simulink model "TrailerSoftware"  (R2019b)
settings: Solver=FixedStepDiscrete  StartTime=0.0  StopTime=inf  FixedStep=update  RelTol=1e-3  EnableMultiTasking=on
values from neighbouring files (symbols this model uses):
  countmax1 = 2500    [ProductionMfile.m]
  countmax2 = 2500    [ProductionMfile.m]
  HeaterIntGain = .0008    (= 0.0008)    [ProductionMfile.m]
  HeatGain = 10    [ProductionMfile.m]
  Intll = 0    [ProductionMfile.m]
  MaxCondPressure = 350    [ProductionMfile.m]
  MinSP = 1    [ProductionMfile.m]
  PostGain100 = 0.0002    [ProductionMfile.m]
  PostGain150 = 0.0005    [ProductionMfile.m]
  PostGain200 = 0.0004    [ProductionMfile.m]
  PostGain300 = 0.0008    [ProductionMfile.m]
  PostInit150 = 12    [ProductionMfile.m]
  PostIntulC = 65    [ProductionMfile.m]
  PostPGain = 0    [ProductionMfile.m]
  PreGain100 = 0.0005    [ProductionMfile.m]
  PreGain150 = 0.0005    [ProductionMfile.m]
  PreGain200 = 0.0003    [ProductionMfile.m]
  PreGain300 = 0.0008    [ProductionMfile.m]
  PreInit150 = 30    [ProductionMfile.m]
  PreIntulC = 65    [ProductionMfile.m]
  PreIntulDH = 65    [ProductionMfile.m]
  PrePGain = 0    [ProductionMfile.m]
  SatPress = [10 20 30 40 50 60 70 80 90 100 110 120 130 140 150 160 170      180 190 200 210 220 230 240 250 260 270 280 290 300 310 320 330      340 350 360 370 380 390 400 410 420 430 440 450 460 470 480 490      500]    [ProductionMfile.m]
  SatTemp = [-29.497 -2.4046 15.401 29.047 40.267 49.88 58.338 65.922 72.819      79.159 85.037 90.526 95.68 100.55 105.16 109.54 113.73 117.73 121.57      125.26 128.82 132.25 135.56 138.77 141.88 144.89 147.82 150.67 153.44      156.15 158.78 161.35 163.85 166.3 168.7 171.04 173.33 175.58 177.77      179.93 182.04 184.11 186.14 188.14 190.09 192.01 193.9 195.75 197.58      199.37]    [ProductionMfile.m]
  SHGain = 2    [ProductionMfile.m]
  SizeCANMatrix = 80    [ProductionMfile.m]
  SizeCOBIDVector = 10    [ProductionMfile.m]
  update = 0.002    [ProductionMfile.m]
undefined symbols (not defined in the file or in its folder): DiscIntNeverNeededParam, PostDGain, PreDGain, Ratio100, Ratio150, Ratio200, Ratio300
libraries: simulink x60, c2837xDlib x35, xpcutilitieslib x24, c2802xlib x8, c280xlib x7, etargetslib x4, svdutilitieslib x2, c2000lib x1
(part 1 of 8)
settings Model: SimulationMode=external  ExtModeTrigDuration=8  Creator=steve  LastModifiedBy=steve
settings SolverCC: AutoInsertRateTranBlk=on
settings DataIOCC: SaveOutput=off  SignalLogging=off  DSMLogging=off  SaveTime=off  ReturnWorkspaceOutputs=off
settings OptimizationCC: DefaultUnderspecifiedDataType=single  EnhancedBackFolding=on  PassReuseOutputArgsAs=Individual arguments  MaxStackSize=1024  OptimizeBlockOrder=speed  DifferentSizesBufferReuse=on  OptimizationCustomize=off  EfficientTunableParamExpr=on
settings DebuggingCC: ParameterTunabilityLossMsg=error
settings HardwareCC: ProdBitPerChar=16  ProdBitPerInt=16  ProdBitPerPointer=32  ProdBitPerSizeT=32  ProdBitPerPtrDiffT=32  ProdLargestAtomicInteger=Integer  ProdLargestAtomicFloat=None  ProdWordSize=16  ProdLongLongMode=on  ProdHWDeviceType=Texas Instruments->C2000
settings SFSimCC: SimCustomSourceCode=src/DisplayFunction.c  SimCustomHeaderCode="#include \"DisplayFunction.h\""  SimUserIncludeDirs=include  MATLABDynamicMemAlloc=off  DefaultCustomCodeFunctionArrayLayout=Row-major  CustomCodeUndefinedFunction=UseInterfaceOnly
settings RTWCC: SystemTargetFile=ert.tlc  HardwareBoard=TI Delfino F28379D LaunchPad  TLCOptions=-aInlineSetEventsForThisBaseRateFcn=TLC_FALSE -aSuppressMultiTaskScheduler=TLC_FALSE -aRateBasedStepFcn=1  TemplateMakefile=ert_default_tmf  Toolchain=Texas Instruments Code Composer Studio (C2000)  IncludeHyperlinkInReport=on
settings CodeAppCC: ForceParamTrailComments=on  IgnoreCustomStorageClasses=off  OperatorAnnotations=on  SimulinkDataObjDesc=on  SFDataObjDesc=on  InsertBlockDesc=on
settings ERTTargetCC: CodeReplacementLibrary=TI C28x  ExtMode=on  ExtModeTransport=3  ExtModeStaticAllocSize=10000  ExtModeMexArgs='127.0.0.1' 0 17725

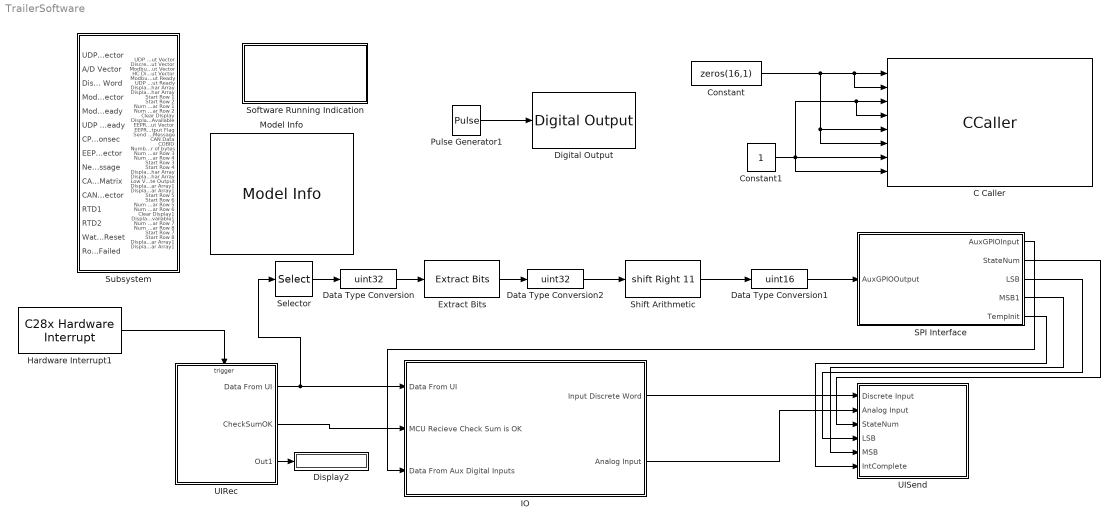
== system TrailerSoftware ==
  C Caller : CCaller  FunctionName=DisplayFunction  PortSpecificationStruct="%)30     .    > X   8    (     @         %    \"     @    !     0         %  0 \"0    $    _    07)G3F%M90  4&]R=$YA;64 4V-O<&4     26YD97@     5'EP90      4VEZ90      27-';&]B86P   X   !     !@    @    $          4    (     0    L    !         !     +    1&ES<&QA>5)O=S$       X   !     !@    @    $          4    (     0    L    !         !     +    1&ES<&QA>5)O=S$       X    X    !@    @    $     ...(+4615 chars)"
  Constant : Constant  Value=zeros(16,1)  OutDataTypeStr=uint8
  Constant1 : Constant  OutDataTypeStr=uint8
  Data Type Conversion : DataTypeConversion  OutDataTypeStr=uint32
  Data Type Conversion1 : DataTypeConversion  OutDataTypeStr=uint16
  Data Type Conversion2 : DataTypeConversion  OutDataTypeStr=uint32
  Digital Output : c2837xDlib/Digital Output  GPIO_Number=GPIO56~GPIO63  GPIO_Bit0=off  GPIO_BIT0_Toggle=off  GPIO_Bit1=off  GPIO_BIT1_Toggle=off  GPIO_Bit2=off  GPIO_BIT2_Toggle=off  GPIO_Bit3=off  GPIO_BIT3_Toggle=off  GPIO_Bit4=off  GPIO_BIT4_Toggle=off  GPIO_Bit5=off  GPIO_BIT5_Toggle=off  GPIO_Bit6=off  GPIO_BIT6_Toggle=off  GPIO_Bit7=on  GPIO_BIT7_Toggle=off
      settings: SourceProductName=Embedded Coder Support Package for Texas Instruments C2000 Processors  SourceProductBaseCode=TIC2000
  Display2 : Display
  Extract Bits : simulink/Logic and Bit Operations/Extract Bits  bitsToExtract=Range of bits  numBits=8  bitIdxRange=[11 18]  outScalingMode=Preserve fixed-point scaling
      settings: SourceProductName=Simulink
  Hardware Interrupt1 : c2000lib/Scheduling/C28x Hardware Interrupt  irqnumbers=[9]  pienumbers=[3]  irqpriorities=[30]  irqpreempts=[1]  showinput=off  dspchiptype=C280X
      settings: SourceProductName=Embedded Coder Support Package for Texas Instruments C2000 Processors  SourceProductBaseCode=TIC2000
  IO : Subsystem
  Model Info : simulink/Model-Wide Utilities/Model Info  Frame=on  DisplayStringWithTags=|  HorizontalTextAlignment=Center  LeftAlignmentValue=0.5
      | Model Info
      | %<Creator>
      | %<ModifiedBy>
      | %<ModelVersion>
      | %<Description>
      | %<LastModifiedBy>
      | %<LastModificationDate>
  Pulse Generator1 : DiscretePulseGenerator  SampleTime=update  VectorParams1D=off
  SPI Interface : Subsystem
  Selector : Selector  InputPortWidth=4  IndexOptions=Index vector (dialog)  Indices=[1]  OutputSizes=1
  Shift Arithmetic : ArithShift  BitShiftNumber=11  BitShiftDirection=Right
  Software Running Indication : Subsystem
  Subsystem : Subsystem
  UIRec : Subsystem
  UISend : Subsystem  TreatAsAtomicUnit=on  SystemSampleTime=.01
  wires:
  IO/1(Input Discrete Word) -> UISend/1(" Discrete Input")
  UIRec/2(CheckSumOK) -> IO/2(MCU Recieve Check Sum is OK)
  UIRec/1(Data From UI) -> Selector/1, IO/1(Data From UI)
  Pulse Generator1/1 -> Digital Output/1
  SPI Interface/1(AuxGPIOInput) -> IO/3(Data From Aux Digital Inputs)
  IO/2(Analog Input) -> UISend/2(Analog Input)
  UIRec/3(Out1) -> Display2/1
  Selector/1 -> Data Type Conversion/1
  Data Type Conversion/1 -> Extract Bits/1
  Extract Bits/1 -> Data Type Conversion2/1
  Shift Arithmetic/1 -> Data Type Conversion1/1
  Data Type Conversion1/1 -> SPI Interface/1(AuxGPIOOutput)
  Data Type Conversion2/1 -> Shift Arithmetic/1
  Hardware Interrupt1/1 -> UIRec/Trigger
  SPI Interface/2(StateNum) -> UISend/3(StateNum)
  SPI Interface/3(LSB) -> UISend/4(LSB)
  SPI Interface/4(MSB1) -> UISend/5(MSB)
  SPI Interface/5(TempInit) -> UISend/6(IntComplete)
  Constant/1 -> C Caller/6, C Caller/5, C Caller/2, C Caller/1
  Constant1/1 -> C Caller/4, C Caller/3, C Caller/8, C Caller/7

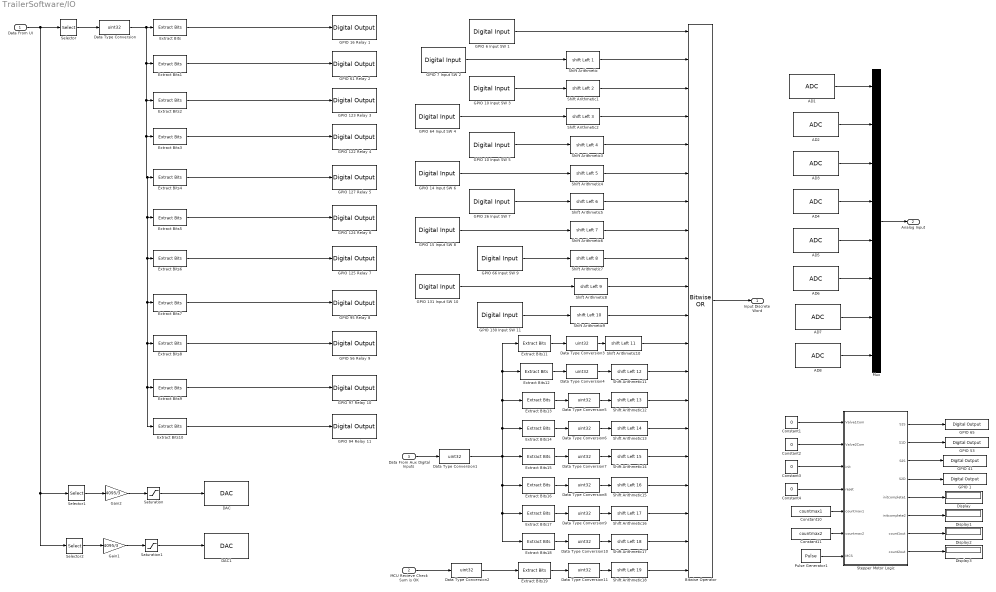
== system TrailerSoftware/IO ==
  Data From UI : Inport
  MCU Recieve Check Sum is OK : Inport  Port=2
  Data From Aux Digital Inputs : Inport  Port=3  OutDataTypeStr=uint16
  AD1 : c2802xlib/ADC  blkParamProc=C2000_Type4  ADCModule=C  samplingMode=Single sample mode  ADCResolution=12-bit (Single-ended input)  useSOC1=SOC0  useSOC2=SOC0_SOC1  SOCAcquisitionWindow=15  SOCTriggerSource=Software  SOCInterruptTrigger=No ADCINT  Ts=update  dType=uint16  postInterrupt=off  interruptSel=ADCINT1  ADCINTContinuous=on  endma=off  chdma=1  conv1=ADCINA0  conv2=ADCINA0 and ADCINB0  conv1_Type4=ADCIN3  conv2_Type4=ADCIN0 and ADCIN1
      settings: SourceProductName=Embedded Coder Support Package for Texas Instruments C2000 Processors
  AD2 : c2802xlib/ADC  blkParamProc=C2000_Type4  ADCModule=B  samplingMode=Single sample mode  ADCResolution=12-bit (Single-ended input)  useSOC1=SOC1  useSOC2=SOC0_SOC1  SOCAcquisitionWindow=15  SOCTriggerSource=Software  SOCInterruptTrigger=No ADCINT  Ts=update  dType=uint16  postInterrupt=off  interruptSel=ADCINT1  ADCINTContinuous=on  endma=off  chdma=1  conv1=ADCINA0  conv2=ADCINA0 and ADCINB0  conv1_Type4=ADCIN3  conv2_Type4=ADCIN0 and ADCIN1
      settings: SourceProductName=Embedded Coder Support Package for Texas Instruments C2000 Processors
  AD3 : c2802xlib/ADC  blkParamProc=C2000_Type4  ADCModule=A  samplingMode=Single sample mode  ADCResolution=12-bit (Single-ended input)  useSOC1=SOC2  useSOC2=SOC0_SOC1  SOCAcquisitionWindow=15  SOCTriggerSource=Software  SOCInterruptTrigger=No ADCINT  Ts=update  dType=uint16  postInterrupt=off  interruptSel=ADCINT1  ADCINTContinuous=on  endma=off  chdma=1  conv1=ADCINA0  conv2=ADCINA0 and ADCINB0  conv1_Type4=ADCIN3  conv2_Type4=ADCIN0 and ADCIN1
      settings: SourceProductName=Embedded Coder Support Package for Texas Instruments C2000 Processors
  AD4 : c2802xlib/ADC  blkParamProc=C2000_Type4  ADCModule=C  samplingMode=Single sample mode  ADCResolution=12-bit (Single-ended input)  useSOC1=SOC3  useSOC2=SOC0_SOC1  SOCAcquisitionWindow=15  SOCTriggerSource=Software  SOCInterruptTrigger=No ADCINT  Ts=update  dType=uint16  postInterrupt=off  interruptSel=ADCINT1  ADCINTContinuous=on  endma=off  chdma=1  conv1=ADCINA0  conv2=ADCINA0 and ADCINB0  conv1_Type4=ADCIN2  conv2_Type4=ADCIN0 and ADCIN1
      settings: SourceProductName=Embedded Coder Support Package for Texas Instruments C2000 Processors
  AD5 : c2802xlib/ADC  blkParamProc=C2000_Type4  ADCModule=B  samplingMode=Single sample mode  ADCResolution=12-bit (Single-ended input)  useSOC1=SOC5  useSOC2=SOC0_SOC1  SOCAcquisitionWindow=15  SOCTriggerSource=Software  SOCInterruptTrigger=No ADCINT  Ts=update  dType=uint16  postInterrupt=off  interruptSel=ADCINT1  ADCINTContinuous=on  endma=off  chdma=1  conv1=ADCINA0  conv2=ADCINA0 and ADCINB0  conv1_Type4=ADCIN2  conv2_Type4=ADCIN0 and ADCIN1
      settings: SourceProductName=Embedded Coder Support Package for Texas Instruments C2000 Processors
  AD6 : c2802xlib/ADC  blkParamProc=C2000_Type4  ADCModule=A  samplingMode=Single sample mode  ADCResolution=12-bit (Single-ended input)  useSOC1=SOC5  useSOC2=SOC0_SOC1  SOCAcquisitionWindow=15  SOCTriggerSource=Software  SOCInterruptTrigger=No ADCINT  Ts=update  dType=uint16  postInterrupt=off  interruptSel=ADCINT1  ADCINTContinuous=on  endma=off  chdma=1  conv1=ADCINA0  conv2=ADCINA0 and ADCINB0  conv1_Type4=ADCIN2  conv2_Type4=ADCIN0 and ADCIN1
      settings: SourceProductName=Embedded Coder Support Package for Texas Instruments C2000 Processors
  AD7 : c2802xlib/ADC  blkParamProc=C2000_Type4  ADCModule=B  samplingMode=Single sample mode  ADCResolution=12-bit (Single-ended input)  useSOC1=SOC6  useSOC2=SOC0_SOC1  SOCAcquisitionWindow=15  SOCTriggerSource=Software  SOCInterruptTrigger=No ADCINT  Ts=update  dType=uint16  postInterrupt=off  interruptSel=ADCINT1  ADCINTContinuous=on  endma=off  chdma=1  conv1=ADCINA0  conv2=ADCINA0 and ADCINB0  conv1_Type4=ADCIN4  conv2_Type4=ADCIN0 and ADCIN1
      settings: SourceProductName=Embedded Coder Support Package for Texas Instruments C2000 Processors
  AD8 : c2802xlib/ADC  blkParamProc=C2000_Type4  ADCModule=C  samplingMode=Single sample mode  ADCResolution=12-bit (Single-ended input)  useSOC1=SOC7  useSOC2=SOC0_SOC1  SOCAcquisitionWindow=15  SOCTriggerSource=Software  SOCInterruptTrigger=No ADCINT  Ts=update  dType=uint16  postInterrupt=off  interruptSel=ADCINT1  ADCINTContinuous=on  endma=off  chdma=1  conv1=ADCINA0  conv2=ADCINA0 and ADCINB0  conv1_Type4=ADCIN5  conv2_Type4=ADCIN0 and ADCIN1
      settings: SourceProductName=Embedded Coder Support Package for Texas Instruments C2000 Processors
  Bitwise Operator : simulink/Logic and Bit Operations/Bitwise Operator  logicop=OR  UseBitMask=off  NumInputPorts=20  BitMask=bin2dec('000000000000')  BitMaskRealWorld=Stored Integer
  Constant{1..4} (4 alike) : Constant  Value=0
  Constant10 : Constant  Value=countmax1
  Constant11 : Constant  Value=countmax2
  DAC : c2837xDlib/DAC  channel=A  saturate=on
      settings: SourceProductName=Embedded Coder Support Package for Texas Instruments C2000 Processors  SourceProductBaseCode=TIC2000
  DAC1 : c2837xDlib/DAC  channel=B  saturate=on
      settings: SourceProductName=Embedded Coder Support Package for Texas Instruments C2000 Processors  SourceProductBaseCode=TIC2000
  Data Type Conversion{,1..11} (12 alike) : DataTypeConversion  OutDataTypeStr=uint32
  Display{,1..3} (4 alike) : Display
  Extract Bits : simulink/Logic and Bit Operations/Extract Bits  bitsToExtract=Range of bits  numBits=8  bitIdxRange=[0]  outScalingMode=Treat bit field as an integer
      settings: SourceProductName=Simulink
  Extract Bits1 : simulink/Logic and Bit Operations/Extract Bits  bitsToExtract=Range of bits  numBits=8  bitIdxRange=[1]  outScalingMode=Treat bit field as an integer
      settings: SourceProductName=Simulink
  Extract Bits10 : simulink/Logic and Bit Operations/Extract Bits  bitsToExtract=Range of bits  numBits=8  bitIdxRange=[10]  outScalingMode=Treat bit field as an integer
      settings: SourceProductName=Simulink
  Extract Bits11 : simulink/Logic and Bit Operations/Extract Bits  bitsToExtract=Range of bits  numBits=8  bitIdxRange=[0]  outScalingMode=Treat bit field as an integer
      settings: SourceProductName=Simulink
  Extract Bits12 : simulink/Logic and Bit Operations/Extract Bits  bitsToExtract=Range of bits  numBits=8  bitIdxRange=[1]  outScalingMode=Treat bit field as an integer
      settings: SourceProductName=Simulink
  Extract Bits13 : simulink/Logic and Bit Operations/Extract Bits  bitsToExtract=Range of bits  numBits=8  bitIdxRange=[2]  outScalingMode=Treat bit field as an integer
      settings: SourceProductName=Simulink
  Extract Bits14 : simulink/Logic and Bit Operations/Extract Bits  bitsToExtract=Range of bits  numBits=8  bitIdxRange=[3]  outScalingMode=Treat bit field as an integer
      settings: SourceProductName=Simulink
  Extract Bits15 : simulink/Logic and Bit Operations/Extract Bits  bitsToExtract=Range of bits  numBits=8  bitIdxRange=[4]  outScalingMode=Treat bit field as an integer
      settings: SourceProductName=Simulink
  Extract Bits16 : simulink/Logic and Bit Operations/Extract Bits  bitsToExtract=Range of bits  numBits=8  bitIdxRange=[5]  outScalingMode=Treat bit field as an integer
      settings: SourceProductName=Simulink
  Extract Bits17 : simulink/Logic and Bit Operations/Extract Bits  bitsToExtract=Range of bits  numBits=8  bitIdxRange=[6]  outScalingMode=Treat bit field as an integer
      settings: SourceProductName=Simulink
  Extract Bits18 : simulink/Logic and Bit Operations/Extract Bits  bitsToExtract=Range of bits  numBits=8  bitIdxRange=[7]  outScalingMode=Treat bit field as an integer
      settings: SourceProductName=Simulink
  Extract Bits19 : simulink/Logic and Bit Operations/Extract Bits  bitsToExtract=Range of bits  numBits=8  bitIdxRange=[0]  outScalingMode=Treat bit field as an integer
      settings: SourceProductName=Simulink
  Extract Bits2 : simulink/Logic and Bit Operations/Extract Bits  bitsToExtract=Range of bits  numBits=8  bitIdxRange=[2]  outScalingMode=Treat bit field as an integer
      settings: SourceProductName=Simulink
  Extract Bits3 : simulink/Logic and Bit Operations/Extract Bits  bitsToExtract=Range of bits  numBits=8  bitIdxRange=[3]  outScalingMode=Treat bit field as an integer
      settings: SourceProductName=Simulink
  Extract Bits4 : simulink/Logic and Bit Operations/Extract Bits  bitsToExtract=Range of bits  numBits=8  bitIdxRange=[4]  outScalingMode=Treat bit field as an integer
      settings: SourceProductName=Simulink
  Extract Bits5 : simulink/Logic and Bit Operations/Extract Bits  bitsToExtract=Range of bits  numBits=8  bitIdxRange=[5]  outScalingMode=Treat bit field as an integer
      settings: SourceProductName=Simulink
  Extract Bits6 : simulink/Logic and Bit Operations/Extract Bits  bitsToExtract=Range of bits  numBits=8  bitIdxRange=[6]  outScalingMode=Treat bit field as an integer
      settings: SourceProductName=Simulink
  Extract Bits7 : simulink/Logic and Bit Operations/Extract Bits  bitsToExtract=Range of bits  numBits=8  bitIdxRange=[7]  outScalingMode=Treat bit field as an integer
      settings: SourceProductName=Simulink
  Extract Bits8 : simulink/Logic and Bit Operations/Extract Bits  bitsToExtract=Range of bits  numBits=8  bitIdxRange=[8]  outScalingMode=Treat bit field as an integer
      settings: SourceProductName=Simulink
  Extract Bits9 : simulink/Logic and Bit Operations/Extract Bits  bitsToExtract=Range of bits  numBits=8  bitIdxRange=[9]  outScalingMode=Treat bit field as an integer
      settings: SourceProductName=Simulink
  GPIO 1 : c2837xDlib/Digital Output  GPIO_Number=GPIO40~GPIO47  GPIO_Bit0=off  GPIO_BIT0_Toggle=off  GPIO_Bit1=on  GPIO_BIT1_Toggle=off  GPIO_Bit2=off  GPIO_BIT2_Toggle=off  GPIO_Bit3=off  GPIO_BIT3_Toggle=off  GPIO_Bit4=off  GPIO_BIT4_Toggle=off  GPIO_Bit5=off  GPIO_BIT5_Toggle=off  GPIO_Bit6=off  GPIO_BIT6_Toggle=off  GPIO_Bit7=off  GPIO_BIT7_Toggle=off
      settings: SourceProductName=Embedded Coder Support Package for Texas Instruments C2000 Processors  SourceProductBaseCode=TIC2000
  GPIO 10 Input SW 3 : c2837xDlib/Digital Input  GPIO_Number=GPIO8~GPIO15  GPIO_Bit0=off  GPIO_Bit1=off  GPIO_Bit2=on  GPIO_Bit3=off  GPIO_Bit4=off  GPIO_Bit5=off  GPIO_Bit6=off  GPIO_Bit7=off  sampleTime=update  dataType=uint32  GPIO_Bit0_Qualification=Sync to SYSCLKOUT  GPIO_Bit1_Qualification=Sync to SYSCLKOUT  GPIO_Bit2_Qualification=Sync to SYSCLKOUT  GPIO_Bit3_Qualification=Sync to SYSCLKOUT  GPIO_Bit4_Qualification=Sync to SYSCLKOUT  GPIO_Bit5_Qualification=Sync to SYSCLKOUT  GPIO_Bit6_Qualification=Sync to SYSCLKOUT  GPIO_Bit7_Qualification=Sync to SYSCLKOUT  Qualification_Period=-1
      settings: SourceProductName=Embedded Coder Support Package for Texas Instruments C2000 Processors  SourceProductBaseCode=TIC2000
  GPIO 10 Input SW 5 : c2837xDlib/Digital Input  GPIO_Number=GPIO64~GPIO71  GPIO_Bit0=on  GPIO_Bit1=off  GPIO_Bit2=off  GPIO_Bit3=off  GPIO_Bit4=off  GPIO_Bit5=off  GPIO_Bit6=off  GPIO_Bit7=off  sampleTime=update  dataType=uint32  GPIO_Bit0_Qualification=Sync to SYSCLKOUT  GPIO_Bit1_Qualification=Sync to SYSCLKOUT  GPIO_Bit2_Qualification=Sync to SYSCLKOUT  GPIO_Bit3_Qualification=Sync to SYSCLKOUT  GPIO_Bit4_Qualification=Sync to SYSCLKOUT  GPIO_Bit5_Qualification=Sync to SYSCLKOUT  GPIO_Bit6_Qualification=Sync to SYSCLKOUT  GPIO_Bit7_Qualification=Sync to SYSCLKOUT  Qualification_Period=-1
      settings: SourceProductName=Embedded Coder Support Package for Texas Instruments C2000 Processors  SourceProductBaseCode=TIC2000
  GPIO 122 Relay 4 : c2837xDlib/Digital Output  GPIO_Number=GPIO120~GPIO127  GPIO_Bit0=off  GPIO_BIT0_Toggle=off  GPIO_Bit1=off  GPIO_BIT1_Toggle=off  GPIO_Bit2=on  GPIO_BIT2_Toggle=off  GPIO_Bit3=off  GPIO_BIT3_Toggle=off  GPIO_Bit4=off  GPIO_BIT4_Toggle=off  GPIO_Bit5=off  GPIO_BIT5_Toggle=off  GPIO_Bit6=off  GPIO_BIT6_Toggle=off  GPIO_Bit7=off  GPIO_BIT7_Toggle=off
      settings: SourceProductName=Embedded Coder Support Package for Texas Instruments C2000 Processors  SourceProductBaseCode=TIC2000
  GPIO 123 Relay 3 : c2837xDlib/Digital Output  GPIO_Number=GPIO120~GPIO127  GPIO_Bit0=off  GPIO_BIT0_Toggle=off  GPIO_Bit1=off  GPIO_BIT1_Toggle=off  GPIO_Bit2=off  GPIO_BIT2_Toggle=off  GPIO_Bit3=on  GPIO_BIT3_Toggle=off  GPIO_Bit4=off  GPIO_BIT4_Toggle=off  GPIO_Bit5=off  GPIO_BIT5_Toggle=off  GPIO_Bit6=off  GPIO_BIT6_Toggle=off  GPIO_Bit7=off  GPIO_BIT7_Toggle=off
      settings: SourceProductName=Embedded Coder Support Package for Texas Instruments C2000 Processors  SourceProductBaseCode=TIC2000
  GPIO 124 Relay 6 : c2837xDlib/Digital Output  GPIO_Number=GPIO120~GPIO127  GPIO_Bit0=off  GPIO_BIT0_Toggle=off  GPIO_Bit1=off  GPIO_BIT1_Toggle=off  GPIO_Bit2=off  GPIO_BIT2_Toggle=off  GPIO_Bit3=off  GPIO_BIT3_Toggle=off  GPIO_Bit4=on  GPIO_BIT4_Toggle=off  GPIO_Bit5=off  GPIO_BIT5_Toggle=off  GPIO_Bit6=off  GPIO_BIT6_Toggle=off  GPIO_Bit7=off  GPIO_BIT7_Toggle=off
      settings: SourceProductName=Embedded Coder Support Package for Texas Instruments C2000 Processors  SourceProductBaseCode=TIC2000
  GPIO 125 Relay 7 : c2837xDlib/Digital Output  GPIO_Number=GPIO120~GPIO127  GPIO_Bit0=off  GPIO_BIT0_Toggle=off  GPIO_Bit1=off  GPIO_BIT1_Toggle=off  GPIO_Bit2=off  GPIO_BIT2_Toggle=off  GPIO_Bit3=off  GPIO_BIT3_Toggle=off  GPIO_Bit4=off  GPIO_BIT4_Toggle=off  GPIO_Bit5=on  GPIO_BIT5_Toggle=off  GPIO_Bit6=off  GPIO_BIT6_Toggle=off  GPIO_Bit7=off  GPIO_BIT7_Toggle=off
      settings: SourceProductName=Embedded Coder Support Package for Texas Instruments C2000 Processors  SourceProductBaseCode=TIC2000
  GPIO 127 Relay 5 : c2837xDlib/Digital Output  GPIO_Number=GPIO24~GPIO31  GPIO_Bit0=off  GPIO_BIT0_Toggle=off  GPIO_Bit1=off  GPIO_BIT1_Toggle=off  GPIO_Bit2=off  GPIO_BIT2_Toggle=off  GPIO_Bit3=on  GPIO_BIT3_Toggle=off  GPIO_Bit4=off  GPIO_BIT4_Toggle=off  GPIO_Bit5=off  GPIO_BIT5_Toggle=off  GPIO_Bit6=off  GPIO_BIT6_Toggle=off  GPIO_Bit7=off  GPIO_BIT7_Toggle=off
      settings: SourceProductName=Embedded Coder Support Package for Texas Instruments C2000 Processors  SourceProductBaseCode=TIC2000
  GPIO 130 Input SW 11 : c2837xDlib/Digital Input  GPIO_Number=GPIO128~GPIO135  GPIO_Bit0=off  GPIO_Bit1=off  GPIO_Bit2=on  GPIO_Bit3=off  GPIO_Bit4=off  GPIO_Bit5=off  GPIO_Bit6=off  GPIO_Bit7=off  sampleTime=update  dataType=uint32  GPIO_Bit0_Qualification=Sync to SYSCLKOUT  GPIO_Bit1_Qualification=Sync to SYSCLKOUT  GPIO_Bit2_Qualification=Sync to SYSCLKOUT  GPIO_Bit3_Qualification=Sync to SYSCLKOUT  GPIO_Bit4_Qualification=Sync to SYSCLKOUT  GPIO_Bit5_Qualification=Sync to SYSCLKOUT  GPIO_Bit6_Qualification=Sync to SYSCLKOUT  GPIO_Bit7_Qualification=Sync to SYSCLKOUT  Qualification_Period=-1
      settings: SourceProductName=Embedded Coder Support Package for Texas Instruments C2000 Processors  SourceProductBaseCode=TIC2000
  GPIO 131 Input SW 10 : c2837xDlib/Digital Input  GPIO_Number=GPIO128~GPIO135  GPIO_Bit0=off  GPIO_Bit1=off  GPIO_Bit2=off  GPIO_Bit3=on  GPIO_Bit4=off  GPIO_Bit5=off  GPIO_Bit6=off  GPIO_Bit7=off  sampleTime=update  dataType=uint32  GPIO_Bit0_Qualification=Sync to SYSCLKOUT  GPIO_Bit1_Qualification=Sync to SYSCLKOUT  GPIO_Bit2_Qualification=Sync to SYSCLKOUT  GPIO_Bit3_Qualification=Sync to SYSCLKOUT  GPIO_Bit4_Qualification=Sync to SYSCLKOUT  GPIO_Bit5_Qualification=Sync to SYSCLKOUT  GPIO_Bit6_Qualification=Sync to SYSCLKOUT  GPIO_Bit7_Qualification=Sync to SYSCLKOUT  Qualification_Period=-1
      settings: SourceProductName=Embedded Coder Support Package for Texas Instruments C2000 Processors  SourceProductBaseCode=TIC2000
  GPIO 14 Input SW 6 : c2837xDlib/Digital Input  GPIO_Number=GPIO8~GPIO15  GPIO_Bit0=off  GPIO_Bit1=off  GPIO_Bit2=off  GPIO_Bit3=off  GPIO_Bit4=off  GPIO_Bit5=off  GPIO_Bit6=on  GPIO_Bit7=off  sampleTime=update  dataType=uint32  GPIO_Bit0_Qualification=Sync to SYSCLKOUT  GPIO_Bit1_Qualification=Sync to SYSCLKOUT  GPIO_Bit2_Qualification=Sync to SYSCLKOUT  GPIO_Bit3_Qualification=Sync to SYSCLKOUT  GPIO_Bit4_Qualification=Sync to SYSCLKOUT  GPIO_Bit5_Qualification=Sync to SYSCLKOUT  GPIO_Bit6_Qualification=Sync to SYSCLKOUT  GPIO_Bit7_Qualification=Sync to SYSCLKOUT  Qualification_Period=-1
      settings: SourceProductName=Embedded Coder Support Package for Texas Instruments C2000 Processors  SourceProductBaseCode=TIC2000
  GPIO 15 Input SW 8 : c2837xDlib/Digital Input  GPIO_Number=GPIO8~GPIO15  GPIO_Bit0=off  GPIO_Bit1=off  GPIO_Bit2=off  GPIO_Bit3=off  GPIO_Bit4=off  GPIO_Bit5=off  GPIO_Bit6=off  GPIO_Bit7=on  sampleTime=update  dataType=uint32  GPIO_Bit0_Qualification=Sync to SYSCLKOUT  GPIO_Bit1_Qualification=Sync to SYSCLKOUT  GPIO_Bit2_Qualification=Sync to SYSCLKOUT  GPIO_Bit3_Qualification=Sync to SYSCLKOUT  GPIO_Bit4_Qualification=Sync to SYSCLKOUT  GPIO_Bit5_Qualification=Sync to SYSCLKOUT  GPIO_Bit6_Qualification=Sync to SYSCLKOUT  GPIO_Bit7_Qualification=Sync to SYSCLKOUT  Qualification_Period=-1
      settings: SourceProductName=Embedded Coder Support Package for Texas Instruments C2000 Processors  SourceProductBaseCode=TIC2000
  GPIO 16 Relay 1 : c2837xDlib/Digital Output  GPIO_Number=GPIO16~GPIO23  GPIO_Bit0=on  GPIO_BIT0_Toggle=off  GPIO_Bit1=off  GPIO_BIT1_Toggle=off  GPIO_Bit2=off  GPIO_BIT2_Toggle=off  GPIO_Bit3=off  GPIO_BIT3_Toggle=off  GPIO_Bit4=off  GPIO_BIT4_Toggle=off  GPIO_Bit5=off  GPIO_BIT5_Toggle=off  GPIO_Bit6=off  GPIO_BIT6_Toggle=off  GPIO_Bit7=off  GPIO_BIT7_Toggle=off
      settings: SourceProductName=Embedded Coder Support Package for Texas Instruments C2000 Processors  SourceProductBaseCode=TIC2000
  GPIO 26 Input SW 7 : c2837xDlib/Digital Input  GPIO_Number=GPIO24~GPIO31  GPIO_Bit0=off  GPIO_Bit1=off  GPIO_Bit2=on  GPIO_Bit3=off  GPIO_Bit4=off  GPIO_Bit5=off  GPIO_Bit6=off  GPIO_Bit7=off  sampleTime=update  dataType=uint32  GPIO_Bit0_Qualification=Sync to SYSCLKOUT  GPIO_Bit1_Qualification=Sync to SYSCLKOUT  GPIO_Bit2_Qualification=Sync to SYSCLKOUT  GPIO_Bit3_Qualification=Sync to SYSCLKOUT  GPIO_Bit4_Qualification=Sync to SYSCLKOUT  GPIO_Bit5_Qualification=Sync to SYSCLKOUT  GPIO_Bit6_Qualification=Sync to SYSCLKOUT  GPIO_Bit7_Qualification=Sync to SYSCLKOUT  Qualification_Period=-1
      settings: SourceProductName=Embedded Coder Support Package for Texas Instruments C2000 Processors  SourceProductBaseCode=TIC2000
  GPIO 41 : c2837xDlib/Digital Output  GPIO_Number=GPIO40~GPIO47  GPIO_Bit0=off  GPIO_BIT0_Toggle=off  GPIO_Bit1=on  GPIO_BIT1_Toggle=off  GPIO_Bit2=off  GPIO_BIT2_Toggle=off  GPIO_Bit3=off  GPIO_BIT3_Toggle=off  GPIO_Bit4=off  GPIO_BIT4_Toggle=off  GPIO_Bit5=off  GPIO_BIT5_Toggle=off  GPIO_Bit6=off  GPIO_BIT6_Toggle=off  GPIO_Bit7=off  GPIO_BIT7_Toggle=off
      settings: SourceProductName=Embedded Coder Support Package for Texas Instruments C2000 Processors  SourceProductBaseCode=TIC2000
  "GPIO 53 " : c2837xDlib/Digital Output  GPIO_Number=GPIO48~GPIO55  GPIO_Bit0=off  GPIO_BIT0_Toggle=off  GPIO_Bit1=off  GPIO_BIT1_Toggle=off  GPIO_Bit2=off  GPIO_BIT2_Toggle=off  GPIO_Bit3=off  GPIO_BIT3_Toggle=off  GPIO_Bit4=off  GPIO_BIT4_Toggle=off  GPIO_Bit5=on  GPIO_BIT5_Toggle=off  GPIO_Bit6=off  GPIO_BIT6_Toggle=off  GPIO_Bit7=off  GPIO_BIT7_Toggle=off
      settings: SourceProductName=Embedded Coder Support Package for Texas Instruments C2000 Processors  SourceProductBaseCode=TIC2000
  GPIO 56 Relay 9 : c2837xDlib/Digital Output  GPIO_Number=GPIO56~GPIO63  GPIO_Bit0=on  GPIO_BIT0_Toggle=off  GPIO_Bit1=off  GPIO_BIT1_Toggle=off  GPIO_Bit2=off  GPIO_BIT2_Toggle=off  GPIO_Bit3=off  GPIO_BIT3_Toggle=off  GPIO_Bit4=off  GPIO_BIT4_Toggle=off  GPIO_Bit5=off  GPIO_BIT5_Toggle=off  GPIO_Bit6=off  GPIO_BIT6_Toggle=off  GPIO_Bit7=off  GPIO_BIT7_Toggle=off
      settings: SourceProductName=Embedded Coder Support Package for Texas Instruments C2000 Processors  SourceProductBaseCode=TIC2000
  GPIO 6 Input SW 1 : c2837xDlib/Digital Input  GPIO_Number=GPIO0~GPIO7  GPIO_Bit0=off  GPIO_Bit1=off  GPIO_Bit2=off  GPIO_Bit3=off  GPIO_Bit4=off  GPIO_Bit5=off  GPIO_Bit6=on  GPIO_Bit7=off  sampleTime=update  dataType=uint32  GPIO_Bit0_Qualification=Sync to SYSCLKOUT  GPIO_Bit1_Qualification=Sync to SYSCLKOUT  GPIO_Bit2_Qualification=Sync to SYSCLKOUT  GPIO_Bit3_Qualification=Sync to SYSCLKOUT  GPIO_Bit4_Qualification=Sync to SYSCLKOUT  GPIO_Bit5_Qualification=Sync to SYSCLKOUT  GPIO_Bit6_Qualification=Sync to SYSCLKOUT  GPIO_Bit7_Qualification=Sync to SYSCLKOUT  Qualification_Period=-1
      settings: SourceProductName=Embedded Coder Support Package for Texas Instruments C2000 Processors  SourceProductBaseCode=TIC2000
  GPIO 61 Relay 2 : c2837xDlib/Digital Output  GPIO_Number=GPIO56~GPIO63  GPIO_Bit0=off  GPIO_BIT0_Toggle=off  GPIO_Bit1=off  GPIO_BIT1_Toggle=off  GPIO_Bit2=off  GPIO_BIT2_Toggle=off  GPIO_Bit3=off  GPIO_BIT3_Toggle=off  GPIO_Bit4=off  GPIO_BIT4_Toggle=off  GPIO_Bit5=on  GPIO_BIT5_Toggle=off  GPIO_Bit6=off  GPIO_BIT6_Toggle=off  GPIO_Bit7=off  GPIO_BIT7_Toggle=off
      settings: SourceProductName=Embedded Coder Support Package for Texas Instruments C2000 Processors  SourceProductBaseCode=TIC2000
  GPIO 64 Input SW 4 : c2837xDlib/Digital Input  GPIO_Number=GPIO8~GPIO15  GPIO_Bit0=off  GPIO_Bit1=off  GPIO_Bit2=off  GPIO_Bit3=on  GPIO_Bit4=off  GPIO_Bit5=off  GPIO_Bit6=off  GPIO_Bit7=off  sampleTime=update  dataType=uint32  GPIO_Bit0_Qualification=Sync to SYSCLKOUT  GPIO_Bit1_Qualification=Sync to SYSCLKOUT  GPIO_Bit2_Qualification=Sync to SYSCLKOUT  GPIO_Bit3_Qualification=Sync to SYSCLKOUT  GPIO_Bit4_Qualification=Sync to SYSCLKOUT  GPIO_Bit5_Qualification=Sync to SYSCLKOUT  GPIO_Bit6_Qualification=Sync to SYSCLKOUT  GPIO_Bit7_Qualification=Sync to SYSCLKOUT  Qualification_Period=-1
      settings: SourceProductName=Embedded Coder Support Package for Texas Instruments C2000 Processors  SourceProductBaseCode=TIC2000
  GPIO 65 : c2837xDlib/Digital Output  GPIO_Number=GPIO64~GPIO71  GPIO_Bit0=off  GPIO_BIT0_Toggle=off  GPIO_Bit1=on  GPIO_BIT1_Toggle=off  GPIO_Bit2=off  GPIO_BIT2_Toggle=off  GPIO_Bit3=off  GPIO_BIT3_Toggle=off  GPIO_Bit4=off  GPIO_BIT4_Toggle=off  GPIO_Bit5=off  GPIO_BIT5_Toggle=off  GPIO_Bit6=off  GPIO_BIT6_Toggle=off  GPIO_Bit7=off  GPIO_BIT7_Toggle=off
      settings: SourceProductName=Embedded Coder Support Package for Texas Instruments C2000 Processors  SourceProductBaseCode=TIC2000
  GPIO 66 Input SW 9 : c2837xDlib/Digital Input  GPIO_Number=GPIO64~GPIO71  GPIO_Bit0=off  GPIO_Bit1=off  GPIO_Bit2=on  GPIO_Bit3=off  GPIO_Bit4=off  GPIO_Bit5=off  GPIO_Bit6=off  GPIO_Bit7=off  sampleTime=update  dataType=uint32  GPIO_Bit0_Qualification=Sync to SYSCLKOUT  GPIO_Bit1_Qualification=Sync to SYSCLKOUT  GPIO_Bit2_Qualification=Sync to SYSCLKOUT  GPIO_Bit3_Qualification=Sync to SYSCLKOUT  GPIO_Bit4_Qualification=Sync to SYSCLKOUT  GPIO_Bit5_Qualification=Sync to SYSCLKOUT  GPIO_Bit6_Qualification=Sync to SYSCLKOUT  GPIO_Bit7_Qualification=Sync to SYSCLKOUT  Qualification_Period=-1
      settings: SourceProductName=Embedded Coder Support Package for Texas Instruments C2000 Processors  SourceProductBaseCode=TIC2000
  GPIO 7 Input SW 2 : c2837xDlib/Digital Input  GPIO_Number=GPIO0~GPIO7  GPIO_Bit0=off  GPIO_Bit1=off  GPIO_Bit2=off  GPIO_Bit3=off  GPIO_Bit4=off  GPIO_Bit5=off  GPIO_Bit6=off  GPIO_Bit7=on  sampleTime=update  dataType=uint32  GPIO_Bit0_Qualification=Sync to SYSCLKOUT  GPIO_Bit1_Qualification=Sync to SYSCLKOUT  GPIO_Bit2_Qualification=Sync to SYSCLKOUT  GPIO_Bit3_Qualification=Sync to SYSCLKOUT  GPIO_Bit4_Qualification=Sync to SYSCLKOUT  GPIO_Bit5_Qualification=Sync to SYSCLKOUT  GPIO_Bit6_Qualification=Sync to SYSCLKOUT  GPIO_Bit7_Qualification=Sync to SYSCLKOUT  Qualification_Period=-1
      settings: SourceProductName=Embedded Coder Support Package for Texas Instruments C2000 Processors  SourceProductBaseCode=TIC2000
  GPIO 94 Relay 11 : c2837xDlib/Digital Output  GPIO_Number=GPIO88~GPIO95  GPIO_Bit0=off  GPIO_BIT0_Toggle=off  GPIO_Bit1=off  GPIO_BIT1_Toggle=off  GPIO_Bit2=off  GPIO_BIT2_Toggle=off  GPIO_Bit3=off  GPIO_BIT3_Toggle=off  GPIO_Bit4=off  GPIO_BIT4_Toggle=off  GPIO_Bit5=off  GPIO_BIT5_Toggle=off  GPIO_Bit6=on  GPIO_BIT6_Toggle=off  GPIO_Bit7=off  GPIO_BIT7_Toggle=off
      settings: SourceProductName=Embedded Coder Support Package for Texas Instruments C2000 Processors  SourceProductBaseCode=TIC2000
  GPIO 95 Relay 8 : c2837xDlib/Digital Output  GPIO_Number=GPIO88~GPIO95  GPIO_Bit0=off  GPIO_BIT0_Toggle=off  GPIO_Bit1=off  GPIO_BIT1_Toggle=off  GPIO_Bit2=off  GPIO_BIT2_Toggle=off  GPIO_Bit3=off  GPIO_BIT3_Toggle=off  GPIO_Bit4=off  GPIO_BIT4_Toggle=off  GPIO_Bit5=off  GPIO_BIT5_Toggle=off  GPIO_Bit6=off  GPIO_BIT6_Toggle=off  GPIO_Bit7=on  GPIO_BIT7_Toggle=off
      settings: SourceProductName=Embedded Coder Support Package for Texas Instruments C2000 Processors  SourceProductBaseCode=TIC2000
  GPIO 97 Relay 10 : c2837xDlib/Digital Output  GPIO_Number=GPIO96~GPIO103  GPIO_Bit0=off  GPIO_BIT0_Toggle=off  GPIO_Bit1=on  GPIO_BIT1_Toggle=off  GPIO_Bit2=off  GPIO_BIT2_Toggle=off  GPIO_Bit3=off  GPIO_BIT3_Toggle=off  GPIO_Bit4=off  GPIO_BIT4_Toggle=off  GPIO_Bit5=off  GPIO_BIT5_Toggle=off  GPIO_Bit6=off  GPIO_BIT6_Toggle=off  GPIO_Bit7=off  GPIO_BIT7_Toggle=off
      settings: SourceProductName=Embedded Coder Support Package for Texas Instruments C2000 Processors  SourceProductBaseCode=TIC2000
  Gain1 : Gain  Gain=4095/3
  Gain2 : Gain  Gain=4095/3
  Mux : Mux  Inputs=8
  Pulse Generator1 : DiscretePulseGenerator  Period=4  SampleTime=update
  Saturation : Saturate  UpperLimit=4095  LowerLimit=0
  Saturation1 : Saturate  UpperLimit=4095  LowerLimit=0
  Selector : Selector  InputPortWidth=4  IndexOptions=Index vector (dialog)  Indices=[1]  OutputSizes=1
  Selector1 : Selector  InputPortWidth=4  IndexOptions=Index vector (dialog)  Indices=[2]  OutputSizes=1
  Selector2 : Selector  InputPortWidth=4  IndexOptions=Index vector (dialog)  Indices=[3]  OutputSizes=1
  Shift Arithmetic : ArithShift  BitShiftNumber=1  BitShiftDirection=Left
  Shift Arithmetic1 : ArithShift  BitShiftNumber=2  BitShiftDirection=Left
  Shift Arithmetic10 : ArithShift  BitShiftNumber=11  BitShiftDirection=Left
  Shift Arithmetic11 : ArithShift  BitShiftNumber=12  BitShiftDirection=Left
  Shift Arithmetic12 : ArithShift  BitShiftNumber=13  BitShiftDirection=Left
  Shift Arithmetic13 : ArithShift  BitShiftNumber=14  BitShiftDirection=Left
  Shift Arithmetic14 : ArithShift  BitShiftNumber=15  BitShiftDirection=Left
  Shift Arithmetic15 : ArithShift  BitShiftNumber=16  BitShiftDirection=Left
  Shift Arithmetic16 : ArithShift  BitShiftNumber=17  BitShiftDirection=Left
  Shift Arithmetic17 : ArithShift  BitShiftNumber=18  BitShiftDirection=Left
  Shift Arithmetic18 : ArithShift  BitShiftNumber=19  BitShiftDirection=Left
  Shift Arithmetic2 : ArithShift  BitShiftNumber=3  BitShiftDirection=Left
  Shift Arithmetic3 : ArithShift  BitShiftNumber=4  BitShiftDirection=Left
  Shift Arithmetic4 : ArithShift  BitShiftNumber=5  BitShiftDirection=Left
  Shift Arithmetic5 : ArithShift  BitShiftNumber=6  BitShiftDirection=Left
  Shift Arithmetic6 : ArithShift  BitShiftNumber=7  BitShiftDirection=Left
  Shift Arithmetic7 : ArithShift  BitShiftNumber=8  BitShiftDirection=Left
  Shift Arithmetic8 : ArithShift  BitShiftNumber=9  BitShiftDirection=Left
  Shift Arithmetic9 : ArithShift  BitShiftNumber=10  BitShiftDirection=Left
  Stepper Motor Logic : MATLAB Function  TreatAsAtomicUnit=on
  Input Discrete Word : Outport
  Analog Input : Outport  Port=2  OutDataTypeStr=uint16
  wires:
  Data From UI/1 -> Selector2/1, Selector1/1, Selector/1
  Extract Bits/1 -> GPIO 16 Relay 1/1
  Extract Bits1/1 -> GPIO 61 Relay 2/1
  Extract Bits2/1 -> GPIO 123 Relay 3/1
  Extract Bits3/1 -> GPIO 122 Relay 4/1
  Extract Bits4/1 -> GPIO 127 Relay 5/1
  Extract Bits5/1 -> GPIO 124 Relay 6/1
  Extract Bits6/1 -> GPIO 125 Relay 7/1
  Extract Bits7/1 -> GPIO 95 Relay 8/1
  Extract Bits8/1 -> GPIO 56 Relay 9/1
  Extract Bits9/1 -> GPIO 97 Relay 10/1
  Selector/1 -> Data Type Conversion/1
  Extract Bits10/1 -> GPIO 94 Relay 11/1
  GPIO 7 Input SW 2/1 -> Shift Arithmetic/1
  GPIO 130 Input SW 11/1 -> Shift Arithmetic9/1
  GPIO 131 Input SW 10/1 -> Shift Arithmetic8/1
  GPIO 66 Input SW 9/1 -> Shift Arithmetic7/1
  GPIO 15 Input SW 8/1 -> Shift Arithmetic6/1
  GPIO 26 Input SW 7/1 -> Shift Arithmetic5/1
  GPIO 14 Input SW 6/1 -> Shift Arithmetic4/1
  GPIO 10 Input SW 5/1 -> Shift Arithmetic3/1
  GPIO 64 Input SW 4/1 -> Shift Arithmetic2/1
  GPIO 10 Input SW 3/1 -> Shift Arithmetic1/1
  GPIO 6 Input SW 1/1 -> Bitwise Operator/1
  Bitwise Operator/1 -> Input Discrete Word/1
  Data Type Conversion/1 -> Extract Bits10/1, Extract Bits9/1, Extract Bits8/1, Extract Bits7/1, Extract Bits6/1, Extract Bits5/1, Extract Bits4/1, Extract Bits3/1, Extract Bits2/1, Extract Bits1/1, Extract Bits/1
  Shift Arithmetic/1 -> Bitwise Operator/2
  Shift Arithmetic1/1 -> Bitwise Operator/3
  Shift Arithmetic2/1 -> Bitwise Operator/4
  Shift Arithmetic3/1 -> Bitwise Operator/5
  Shift Arithmetic4/1 -> Bitwise Operator/6
  Shift Arithmetic5/1 -> Bitwise Operator/7
  Shift Arithmetic6/1 -> Bitwise Operator/8
  Shift Arithmetic7/1 -> Bitwise Operator/9
  Shift Arithmetic8/1 -> Bitwise Operator/10
  Shift Arithmetic9/1 -> Bitwise Operator/11
  Extract Bits11/1 -> Data Type Conversion3/1
  Data From Aux Digital Inputs/1 -> Data Type Conversion1/1
  Data Type Conversion1/1 -> Extract Bits14/1, Extract Bits12/1, Extract Bits11/1, Extract Bits13/1, Extract Bits18/1, Extract Bits17/1, Extract Bits16/1, Extract Bits15/1
  Extract Bits12/1 -> Data Type Conversion4/1
  Extract Bits13/1 -> Data Type Conversion5/1
  Extract Bits14/1 -> Data Type Conversion6/1
  Extract Bits15/1 -> Data Type Conversion7/1
  Extract Bits16/1 -> Data Type Conversion8/1
  Extract Bits17/1 -> Data Type Conversion9/1
  Extract Bits18/1 -> Data Type Conversion10/1
  Shift Arithmetic11/1 -> Bitwise Operator/13
  Shift Arithmetic12/1 -> Bitwise Operator/14
  Shift Arithmetic13/1 -> Bitwise Operator/15
  Shift Arithmetic14/1 -> Bitwise Operator/16
  Shift Arithmetic15/1 -> Bitwise Operator/17
  Shift Arithmetic16/1 -> Bitwise Operator/18
  Shift Arithmetic17/1 -> Bitwise Operator/19
  Shift Arithmetic18/1 -> Bitwise Operator/20
  MCU Recieve Check Sum is OK/1 -> Data Type Conversion2/1
  Extract Bits19/1 -> Data Type Conversion11/1
  Data Type Conversion2/1 -> Extract Bits19/1
  Shift Arithmetic10/1 -> Bitwise Operator/12
  AD3/1 -> Mux/3
  AD4/1 -> Mux/4
  AD6/1 -> Mux/6
  AD1/1 -> Mux/1
  AD2/1 -> Mux/2
  AD5/1 -> Mux/5
  Mux/1 -> Analog Input/1
  AD7/1 -> Mux/7
  AD8/1 -> Mux/8
  Selector1/1 -> Gain2/1
  Selector2/1 -> Gain1/1
  Gain2/1 -> Saturation/1
  Gain1/1 -> Saturation1/1
  Saturation/1 -> DAC/1
  Saturation1/1 -> DAC1/1
  Constant11/1 -> Stepper Motor Logic/6(countmax2)
  Stepper Motor Logic/3(S2S) -> GPIO 41/1
  Stepper Motor Logic/6(initcomplete2) -> Display1/1
  Stepper Motor Logic/5(initcomplete1) -> Display/1
  Constant10/1 -> Stepper Motor Logic/5(countmax1)
  Stepper Motor Logic/1(S1S) -> GPIO 65/1
  Constant4/1 -> Stepper Motor Logic/4(reset)
  Stepper Motor Logic/8(count2out) -> Display3/1
  Stepper Motor Logic/2(S1D) -> "GPIO 53 "/1
  Constant1/1 -> Stepper Motor Logic/1(Valve1Com)
  Stepper Motor Logic/4(S2D) -> GPIO 1/1
  Constant2/1 -> Stepper Motor Logic/2(Valve2Com)
  Constant3/1 -> Stepper Motor Logic/3(init)
  Pulse Generator1/1 -> Stepper Motor Logic/7(MCS)
  Stepper Motor Logic/7(count1out) -> Display2/1
  Data Type Conversion3/1 -> Shift Arithmetic10/1
  Data Type Conversion4/1 -> Shift Arithmetic11/1
  Data Type Conversion5/1 -> Shift Arithmetic12/1
  Data Type Conversion6/1 -> Shift Arithmetic13/1
  Data Type Conversion7/1 -> Shift Arithmetic14/1
  Data Type Conversion8/1 -> Shift Arithmetic15/1
  Data Type Conversion9/1 -> Shift Arithmetic16/1
  Data Type Conversion10/1 -> Shift Arithmetic17/1
  Data Type Conversion11/1 -> Shift Arithmetic18/1

== system TrailerSoftware/SPI Interface ==
  AuxGPIOOutput : Inport  OutDataTypeStr=uint16
  Chart : Stateflow chart  BlockKeywords=__PRM__SERIALIZED__DATA__:Stateflow Chart,Stateflow Diagram  TreatAsAtomicUnit=on
  Terminator : Terminator
  Terminator1 : Terminator
  Terminator2 : Terminator
  AuxGPIOInput : Outport  OutDataTypeStr=uint16
  StateNum : Outport  Port=2
  LSB : Outport  Port=3  OutDataTypeStr=uint16
  MSB1 : Outport  Port=4  OutDataTypeStr=uint16
  TempInit : Outport  Port=5  OutDataTypeStr=uint16
  wires:
  AuxGPIOOutput/1 -> Chart/1(AuxGPIOOutput)
  Chart/3(TFault1) -> Terminator/1
  Chart/4(TOut1) -> Terminator2/1
  Chart/1(AuxGPIOInput) -> AuxGPIOInput/1
  Chart/5(StateNum) -> StateNum/1
  Chart/2(value) -> Terminator1/1
  Chart/6(LSB) -> LSB/1
  Chart/7(MSB) -> MSB1/1
  Chart/8(TempsInitComplete) -> TempInit/1

== system TrailerSoftware/Software Running Indication ==
  Digital Output : c2837xDlib/Digital Output  GPIO_Number=GPIO24~GPIO31  GPIO_Bit0=off  GPIO_BIT0_Toggle=off  GPIO_Bit1=off  GPIO_BIT1_Toggle=off  GPIO_Bit2=off  GPIO_BIT2_Toggle=off  GPIO_Bit3=off  GPIO_BIT3_Toggle=off  GPIO_Bit4=off  GPIO_BIT4_Toggle=off  GPIO_Bit5=off  GPIO_BIT5_Toggle=off  GPIO_Bit6=off  GPIO_BIT6_Toggle=off  GPIO_Bit7=on  GPIO_BIT7_Toggle=off
      settings: SourceProductName=Embedded Coder Support Package for Texas Instruments C2000 Processors  SourceProductBaseCode=TIC2000
  Pulse Generator1 : DiscretePulseGenerator  Period=20  PulseWidth=10  SampleTime=0.05  VectorParams1D=off
  wires:
  Pulse Generator1/1 -> Digital Output/1
